simulink model "P2D_JustPlantStep_NoNoise_NoVarInput"  (R2022a)
settings: Solver=VariableStepAuto  StartTime=0.0  StopTime=1  RelTol=1e-3
settings Model: Creator=tyevans  LastModifiedBy=tyevans

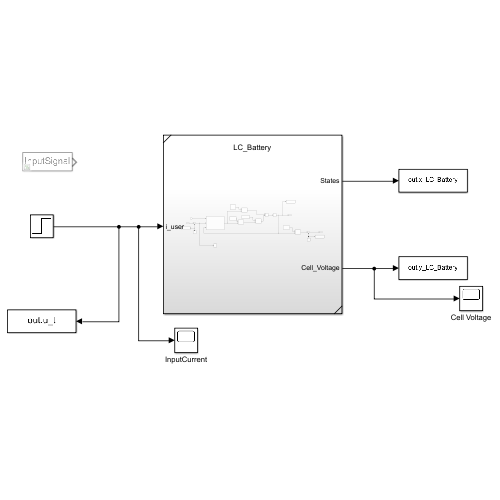
[thumbnail: Simulink's stored preview of the top-level diagram]
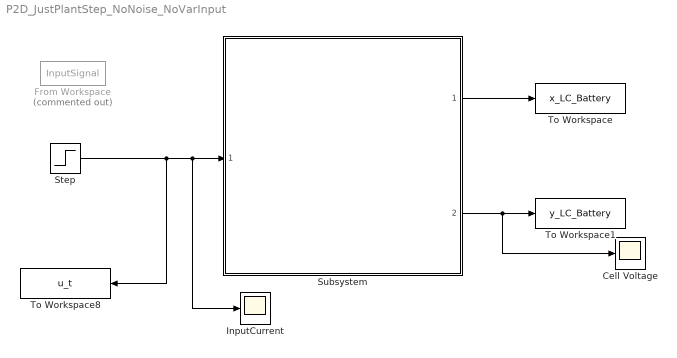
== system P2D_JustPlantStep_NoNoise_NoVarInput ==
  Cell Voltage : Scope
  From Workspace : FromWorkspace  Commented=on  VariableName=InputSignal  Interpolate=off  OutputAfterFinalValue=Setting to zero
  InputCurrent : Scope
  Step : Step  Time=2  SampleTime=0
  Subsystem : Subsystem  ReferencedSubsystem=LC_Battery
  To Workspace : ToWorkspace  VariableName=x_LC_Battery  SaveFormat=Structure With Time  SampleTime=-1
  To Workspace1 : ToWorkspace  VariableName=y_LC_Battery  SaveFormat=Structure With Time  SampleTime=-1
  To Workspace8 : ToWorkspace  VariableName=u_t  SaveFormat=Structure With Time  SampleTime=-1
  wires:
  Subsystem/1 -> To Workspace/1
  Subsystem/2 -> To Workspace1/1, Cell Voltage/1
  Step/1 -> To Workspace8/1, InputCurrent/1, Subsystem/1
